simulink model "bandpassFilter"  (R2023a)
settings: Solver=VariableStepAuto  StartTime=0.0  StopTime=1  RelTol=1e-9
model workspace (MAT data in the model file):
  Q = 10
  omegac = 9424.77796077
settings Model: ParameterArgumentNames=Q,omegac  Creator=mcconncm  LastModifiedBy=mcconncm

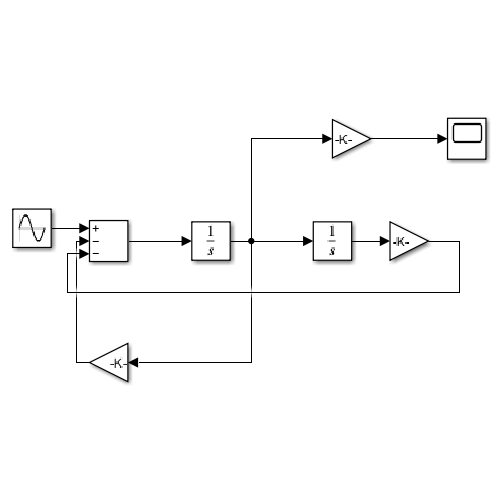
[thumbnail: Simulink's stored preview of the top-level diagram]
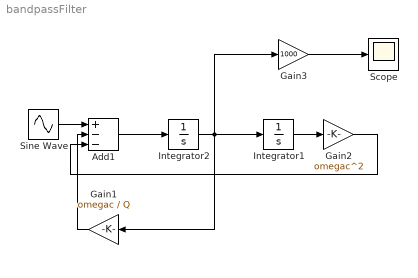
== system bandpassFilter ==
  Add1 : Sum  Inputs=+--
  Gain1 : Gain  Gain=omegac / Q
  Gain2 : Gain  Gain=omegac^2
  Gain3 : Gain  Gain=1000
  Integrator1 : Integrator
  Integrator2 : Integrator
  Scope : Scope
  Sine Wave : Sin  Frequency=1500*2*pi  SampleTime=0
  wires:
  Add1/1 -> Integrator2/1
  Gain1/1 -> Add1/2
  Integrator2/1 -> Gain3/1, Gain1/1, Integrator1/1
  Sine Wave/1 -> Add1/1
  Integrator1/1 -> Gain2/1
  Gain2/1 -> Add1/3
  Gain3/1 -> Scope/1
